simulink model "MNR"  (R2019b)
settings: Solver=FixedStepDiscrete  StartTime=0.0  StopTime=stop_time  RelTol=1e-3
InitFcn:
  | sm_callback_init
StopFcn:
  | sm_callback_stop
values from neighbouring files (symbols this model uses):
  mp = sm_init_avalon_signals(mp)    [sm_callback_init.m]    (also in sm_callback_stop.m = sm_stop_verify(mp))
libraries: simulink x1
settings Model: Creator=Ross  LastModifiedBy=trevor
settings DataIOCC: ReturnWorkspaceOutputs=off
settings OptimizationCC: BlockReduction=off  ConditionallyExecuteInputs=off  DefaultParameterBehavior=Inlined
settings DebuggingCC: ReadBeforeWriteMsg=DisableAll  WriteAfterWriteMsg=DisableAll  WriteAfterReadMsg=DisableAll  AlgebraicLoopMsg=error  MultiTaskDSMMsg=none  SingleTaskRateTransMsg=error  PregeneratedLibrarySubsystemCodeDiagnostic=none  ArithmeticOperatorsInVariantConditions=warning
settings HardwareCC: ProdBitPerPointer=32  ProdBitPerSizeT=32  ProdBitPerPtrDiffT=32  ProdLargestAtomicFloat=None  ProdIntDivRoundTo=Undefined  ProdEndianess=Unspecified  ProdWordSize=32  ProdHWDeviceType=ASIC/FPGA->ASIC/FPGA  TargetBitPerLong=64  TargetBitPerPointer=64  TargetBitPerSizeT=64  TargetBitPerPtrDiffT=64  TargetLongLongMode=on  TargetIntDivRoundTo=Zero  TargetEndianess=LittleEndian  TargetWordSize=64  TargetHWDeviceType=Custom Processor->MATLAB Host Computer  ProdEqTarget=off
settings ModelReferenceCC: UpdateModelReferenceTargets=IfOutOfDate
settings SFSimCC: SFSimEcho=off  SimUseLocalCustomCode=off  CustomCodeUndefinedFunction=UseInterfaceOnly
settings RTWCC: RTWUseLocalCustomCode=off

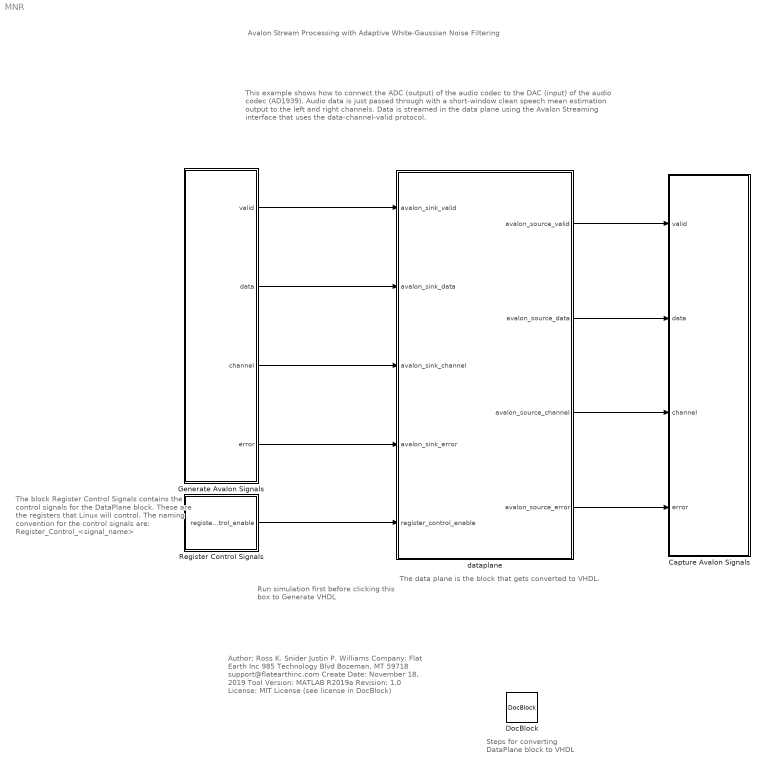
== system MNR ==
  note: The data plane is the block that gets converted to VHDL.
  note: Author:          Ross K. Snider
      |                      Justin P. Williams
      | Company:     Flat Earth Inc
      |                       985 Technology Blvd
      |                       Bozeman, MT 59718
      |                       support@flatearthinc.com
      | Create Date:  November 18, 2019
      | Tool Version:  MATLAB R2019a
      | Revision:        1.0
      | License:          MIT License (see license in DocBlock)
  note: This example shows how to connect the ADC (output) of the audio codec to the DAC (input) of the audio codec (AD1939). Audio data is just passed through with a short-window clean speech mean estimation output to the left and right channels. Data is streamed in the data plane using the Avalon Streaming interface that uses the data-channel-valid protocol.
  note: Steps for converting
      | DataPlane block
      | to VHDL
  note: Avalon Stream Processing
      | with Adaptive White-Gaussian Noise Filtering
  note: Run simulation first
      | before clicking this box to
      | Generate VHDL
  note: The block Register Control Signals contains
      | the control signals for the DataPlane block.
      | These are the registers that Linux will control.
      | The naming convention for the control
      | signals are:  Register_Control_<signal_name>
  Capture Avalon Signals : Subsystem
  DocBlock : simulink/Model-Wide Utilities/DocBlock  DocumentType=HTML
  Generate Avalon Signals : Subsystem
  Register Control Signals : Subsystem
  dataplane : Subsystem  TreatAsAtomicUnit=on
  wires:
  Generate Avalon Signals/2(data) -> dataplane/2(avalon_sink_data)
  Generate Avalon Signals/1(valid) -> dataplane/1(avalon_sink_valid)
  Generate Avalon Signals/3(channel) -> dataplane/3(avalon_sink_channel)
  Generate Avalon Signals/4(error) -> dataplane/4(avalon_sink_error)
  dataplane/2(avalon_source_data) -> Capture Avalon Signals/2(data)
  dataplane/1(avalon_source_valid) -> Capture Avalon Signals/1(valid)
  dataplane/3(avalon_source_channel) -> Capture Avalon Signals/3(channel)
  dataplane/4(avalon_source_error) -> Capture Avalon Signals/4(error)
  Register Control Signals/1(register_control_enable) -> dataplane/5(register_control_enable)

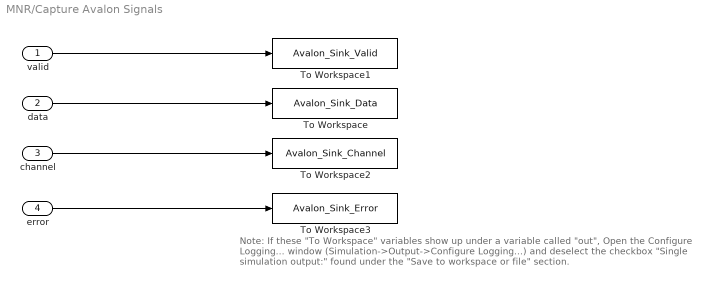
== system MNR/Capture Avalon Signals ==
  note: Note:  If these "To Workspace" variables show up under a variable called "out",
      | Open the Configure Logging... window (Simulation->Output->Configure Logging...)
      | and deselect the checkbox "Single simulation output:" found under the "Save to workspace or file" section.
  valid : Inport
  data : Inport  Port=2
  channel : Inport  Port=3
  error : Inport  Port=4
  To Workspace : ToWorkspace  VariableName=Avalon_Sink_Data  SaveFormat=Timeseries  SampleTime=-1
  To Workspace1 : ToWorkspace  VariableName=Avalon_Sink_Valid  SaveFormat=Timeseries  SampleTime=-1
  To Workspace2 : ToWorkspace  VariableName=Avalon_Sink_Channel  SaveFormat=Timeseries  SampleTime=-1
  To Workspace3 : ToWorkspace  VariableName=Avalon_Sink_Error  SaveFormat=Timeseries  SampleTime=-1
  wires:
  data/1 -> To Workspace/1
  valid/1 -> To Workspace1/1
  error/1 -> To Workspace3/1
  channel/1 -> To Workspace2/1

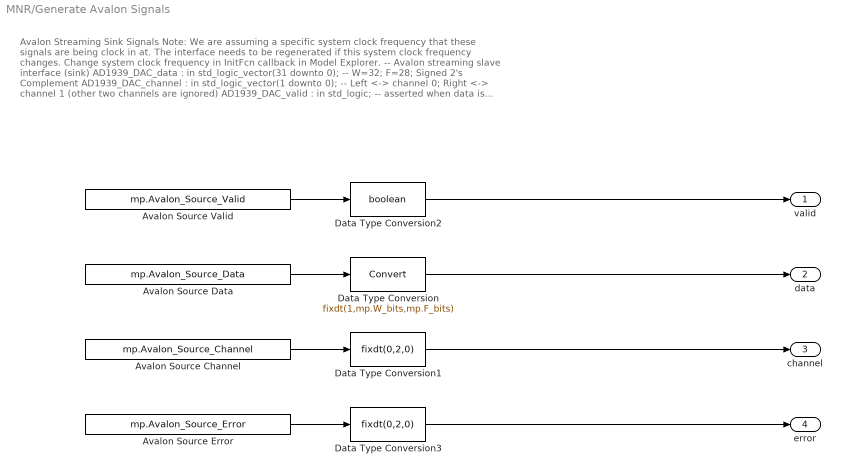
== system MNR/Generate Avalon Signals ==
  note: Avalon Streaming Sink Signals
      | Note: We are assuming a specific system clock frequency that these signals are being clock in at.
      | The interface needs to be regenerated if this system clock frequency changes. Change system clock frequency in InitFcn callback in Model Explorer.
      |
      | -- Avalon streaming slave interface (sink)
      | AD1939_DAC_data : in std_logic_vector(31 downto 0); -- W=32; F=28; Signed 2's Complement
      | AD1939_DAC_channel : in std_logic_vector(1 downto 0); -- Left <-> channel 0; Right <-> channel 1 (other two channels are ignored)
      | AD1939_DAC_valid : in std_logic; -- asserted when data is valid
      | AD1939_DAC_error : in std_logic_vector(1 downto 0) -- error channel is ignored, assumed to be error free at this point
      |
      | For more information on the data-channel-valid protocol, s ee chapter 5 in Intel's Avalon Interfaced Specification (p. 40) at https://www.intel.com/content/dam/www/programmable/us/en/pdfs/literature/manual/mnl_avalon_spec.pdf
  Avalon Source Channel : FromWorkspace  VariableName=mp.Avalon_Source_Channel  OutDataTypeStr=double  SampleTime=mp.Ts_system
  "Avalon Source Data " : FromWorkspace  VariableName=mp.Avalon_Source_Data  OutDataTypeStr=double  SampleTime=mp.Ts_system
  Avalon Source Error : FromWorkspace  VariableName=mp.Avalon_Source_Error  OutDataTypeStr=double  SampleTime=mp.Ts_system
  Avalon Source Valid : FromWorkspace  VariableName=mp.Avalon_Source_Valid  OutDataTypeStr=double  SampleTime=mp.Ts_system
  Data Type Conversion : DataTypeConversion  OutDataTypeStr=fixdt(1,mp.W_bits,mp.F_bits)
  Data Type Conversion1 : DataTypeConversion  OutDataTypeStr=fixdt(0,2,0)
  Data Type Conversion2 : DataTypeConversion  OutDataTypeStr=boolean
  Data Type Conversion3 : DataTypeConversion  OutDataTypeStr=fixdt(0,2,0)
  valid : Outport  VectorParamsAs1DForOutWhenUnconnected=off
  data : Outport  Port=2  VectorParamsAs1DForOutWhenUnconnected=off
  channel : Outport  Port=3  VectorParamsAs1DForOutWhenUnconnected=off
  error : Outport  Port=4  VectorParamsAs1DForOutWhenUnconnected=off
  wires:
  Data Type Conversion1/1 -> channel/1
  Data Type Conversion2/1 -> valid/1
  Avalon Source Error/1 -> Data Type Conversion3/1
  Data Type Conversion/1 -> data/1
  Avalon Source Valid/1 -> Data Type Conversion2/1
  Data Type Conversion3/1 -> error/1
  Avalon Source Channel/1 -> Data Type Conversion1/1
  "Avalon Source Data "/1 -> Data Type Conversion/1

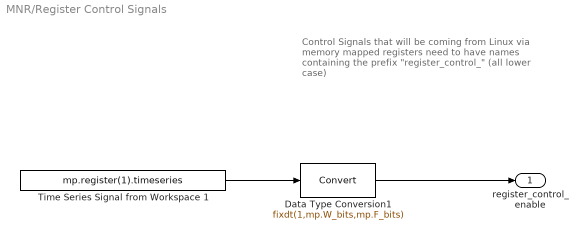
== system MNR/Register Control Signals ==
  note: Control Signals that will be coming from Linux via
      | memory mapped registers need to have names
      | containing the prefix "register_control_"
      | (all lower case)
  Data Type Conversion1 : DataTypeConversion  OutDataTypeStr=fixdt(1,mp.W_bits,mp.F_bits)
  Time Series Signal from Workspace 1 : FromWorkspace  VariableName=mp.register(1).timeseries  OutDataTypeStr=double  SampleTime=mp.Ts_system
  register_control_enable : Outport  VectorParamsAs1DForOutWhenUnconnected=off
  wires:
  Time Series Signal from Workspace 1/1 -> Data Type Conversion1/1
  Data Type Conversion1/1 -> register_control_enable/1

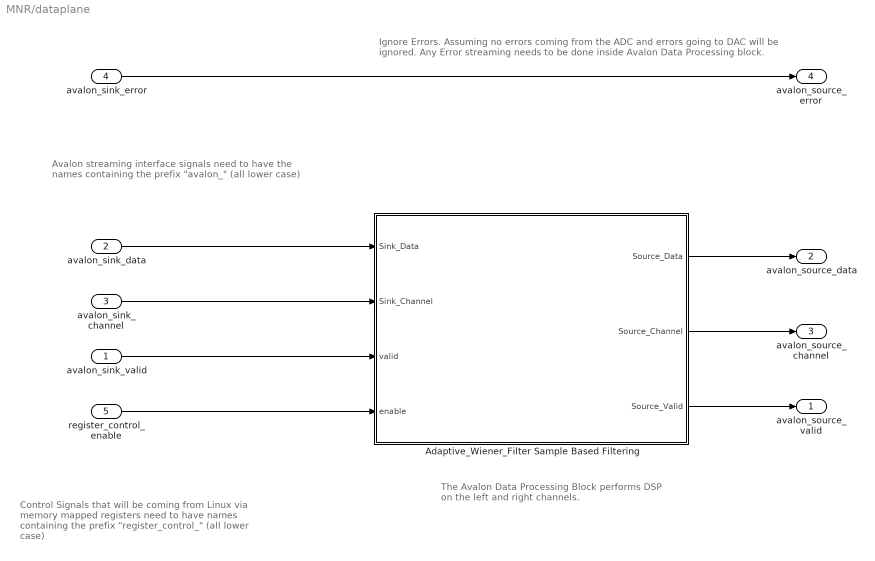
== system MNR/dataplane ==
  note: Control Signals that will be coming from Linux via
      | memory mapped registers need to have names
      | containing the prefix "register_control_"
      | (all lower case)
  note: The Avalon Data Processing Block
      | performs DSP on the left and right channels.
  note: Ignore Errors.
      | Assuming no errors coming from the ADC and errors going to DAC will be ignored.
      | Any Error streaming needs to be done inside Avalon Data Processing block.
  note: Avalon streaming interface signals need to have the
      | names containing the prefix "avalon_"
      | (all lower case)
  avalon_sink_valid : Inport
  avalon_sink_data : Inport  Port=2
  avalon_sink_channel : Inport  Port=3
  avalon_sink_error : Inport  Port=4
  register_control_enable : Inport  Port=5
  Adaptive_Wiener_Filter Sample Based Filtering : Subsystem
  avalon_source_valid : Outport  VectorParamsAs1DForOutWhenUnconnected=off
  avalon_source_data : Outport  Port=2  VectorParamsAs1DForOutWhenUnconnected=off
  avalon_source_channel : Outport  Port=3  VectorParamsAs1DForOutWhenUnconnected=off
  avalon_source_error : Outport  Port=4  VectorParamsAs1DForOutWhenUnconnected=off
  wires:
  avalon_sink_error/1 -> avalon_source_error/1
  Adaptive_Wiener_Filter Sample Based Filtering/1(Source_Data) -> avalon_source_data/1
  avalon_sink_data/1 -> Adaptive_Wiener_Filter Sample Based Filtering/1(Sink_Data)
  Adaptive_Wiener_Filter Sample Based Filtering/2(Source_Channel) -> avalon_source_channel/1
  avalon_sink_channel/1 -> Adaptive_Wiener_Filter Sample Based Filtering/2(Sink_Channel)
  register_control_enable/1 -> Adaptive_Wiener_Filter Sample Based Filtering/4(enable)
  avalon_sink_valid/1 -> Adaptive_Wiener_Filter Sample Based Filtering/3(valid)
  Adaptive_Wiener_Filter Sample Based Filtering/3(Source_Valid) -> avalon_source_valid/1

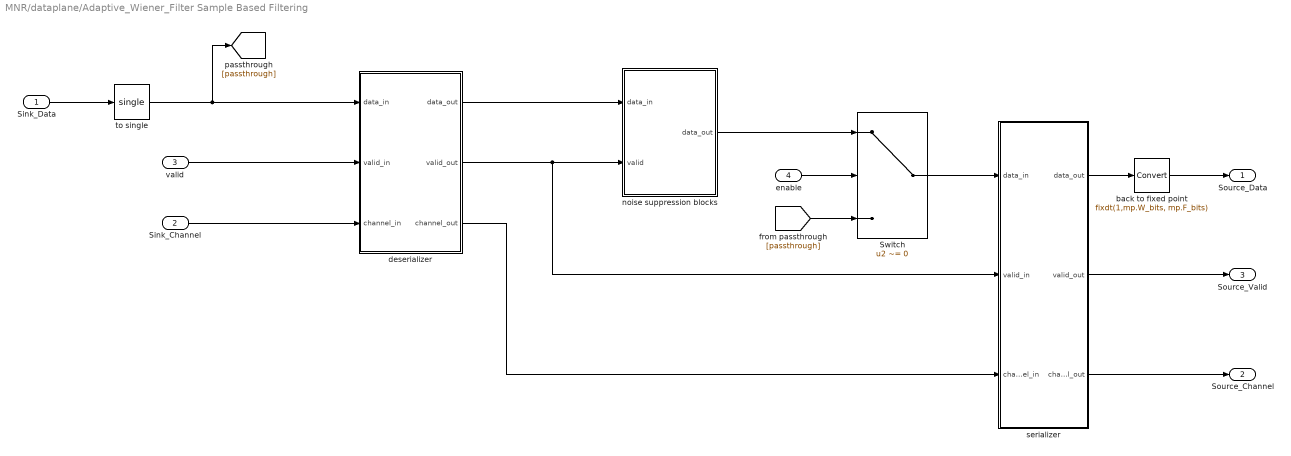
== system MNR/dataplane/Adaptive_Wiener_Filter Sample Based Filtering ==
  Sink_Data : Inport
  Sink_Channel : Inport  Port=2
  valid : Inport  Port=3
  enable : Inport  Port=4
  Switch : Switch  Criteria=u2 ~= 0  Threshold=1
  back to fixed point : DataTypeConversion  OutDataTypeStr=fixdt(1,mp.W_bits, mp.F_bits)  RndMeth=Nearest
  deserializer : MATLAB Function  TreatAsAtomicUnit=on
  noise suppression blocks : Subsystem  TreatAsAtomicUnit=on
  serializer : MATLAB Function  TreatAsAtomicUnit=on
  to single : DataTypeConversion  OutDataTypeStr=single  RndMeth=Nearest
  Source_Data : Outport  InitialOutput=0  VectorParamsAs1DForOutWhenUnconnected=off
  Source_Channel : Outport  Port=2  InitialOutput=0  VectorParamsAs1DForOutWhenUnconnected=off
  Source_Valid : Outport  Port=3  InitialOutput=0  VectorParamsAs1DForOutWhenUnconnected=off
  wires:
  enable/1 -> Switch/2
  to single/1 -> [passthrough], deserializer/1(data_in)
  valid/1 -> deserializer/2(valid_in)
  Sink_Channel/1 -> deserializer/3(channel_in)
  deserializer/2(valid_out) -> serializer/2(valid_in), noise suppression blocks/2(valid)
  deserializer/1(data_out) -> noise suppression blocks/1(data_in)
  noise suppression blocks/1(data_out) -> Switch/1
  [passthrough] -> Switch/3
  Sink_Data/1 -> to single/1
  back to fixed point/1 -> Source_Data/1
  serializer/1(data_out) -> back to fixed point/1
  Switch/1 -> serializer/1(data_in)
  serializer/3(channel_out) -> Source_Channel/1
  serializer/2(valid_out) -> Source_Valid/1
  deserializer/3(channel_out) -> serializer/3(channel_in)

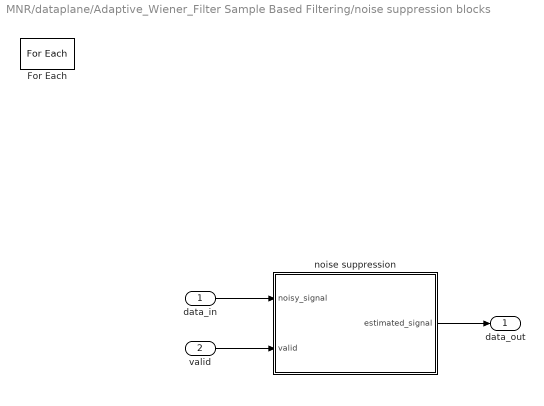
== system MNR/dataplane/Adaptive_Wiener_Filter Sample Based Filtering/noise suppression blocks ==
  data_in : Inport  Partition=on  PartitionDimension=1  PartitionWidth=1  PartitionOffset=0
  valid : Inport  Port=2
  For Each : ForEach  DisableCoverage=on
  noise suppression : Subsystem  TreatAsAtomicUnit=on
  data_out : Outport  ConcatenationDimension=1
  wires:
  noise suppression/1("estimated_signal ") -> data_out/1
  data_in/1 -> noise suppression/1(noisy_signal)
  valid/1 -> noise suppression/2(valid)

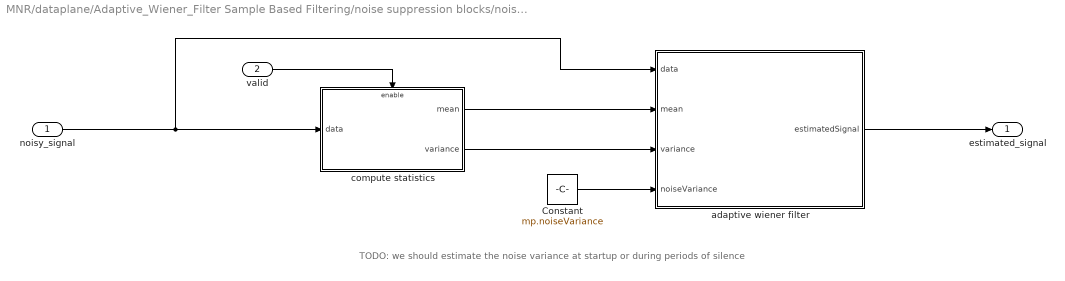
== system MNR/dataplane/Adaptive_Wiener_Filter Sample Based Filtering/noise suppression blocks/noise suppression ==
  note: TODO: we should estimate the noise variance at startup or during periods of silence
  noisy_signal : Inport
  valid : Inport  Port=2
  Constant : Constant  Value=mp.noiseVariance  SampleTime=-1
  adaptive wiener filter : MATLAB Function  TreatAsAtomicUnit=on
  compute statistics : Subsystem
  "estimated_signal " : Outport  InitialOutput=0  VectorParamsAs1DForOutWhenUnconnected=off
  wires:
  compute statistics/2(variance) -> adaptive wiener filter/3(variance)
  compute statistics/1(mean) -> adaptive wiener filter/2(mean)
  noisy_signal/1 -> adaptive wiener filter/1(data), compute statistics/1(data)
  valid/1 -> compute statistics/Enable
  adaptive wiener filter/1(estimatedSignal) -> "estimated_signal "/1
  Constant/1 -> adaptive wiener filter/4(noiseVariance)

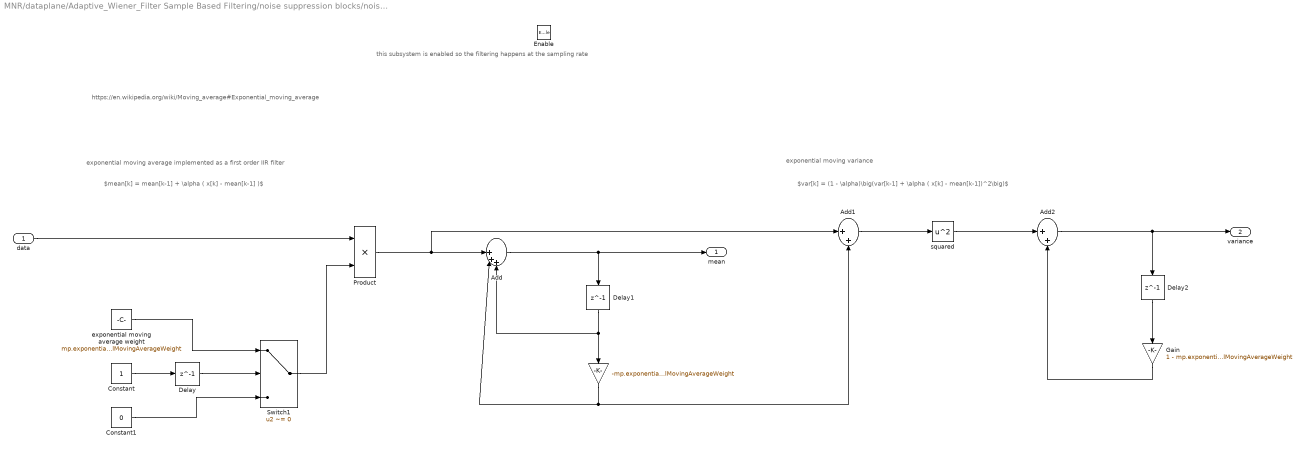
== system MNR/dataplane/Adaptive_Wiener_Filter Sample Based Filtering/noise suppression blocks/noise suppression/compute statistics ==
  note: https://en.wikipedia.org/wiki/Moving_average#Exponential_moving_average
  note: this subsystem is enabled so the filtering happens at the sampling rate
  note: $mean[k] = mean[k-1] + \alpha ( x[k] - mean[k-1] )$
  note: exponential moving variance
  note: exponential moving average implemented as a first order IIR filter
  note: $var[k] = (1 - \alpha)\big(var[k-1] + \alpha ( x[k] - mean[k-1])^2\big)$
  data : Inport
  Enable : EnablePort
  " " : Gain  Gain=-mp.exponentialMovingAverageWeight
  Add : Sum  Inputs=||+++
  Add1 : Sum  Inputs=|++
  Add2 : Sum  Inputs=|++
  Constant : Constant  OutDataTypeStr=boolean
  Constant1 : Constant  Value=0  OutDataTypeStr=single
  Delay : Delay  DelayLength=1  InitialCondition=0
  Delay1 : Delay  DelayLength=1  InitialCondition=0
  Delay2 : Delay  DelayLength=1  InitialCondition=0
  Gain : Gain  Gain=1 - mp.exponentialMovingAverageWeight
  Product : Product
  Switch1 : Switch  Criteria=u2 ~= 0
  exponential moving average weight : Constant  Value=mp.exponentialMovingAverageWeight
  squared : Math  Operator=square  RndMeth=Zero  SaturateOnIntegerOverflow=on
  mean : Outport
  variance : Outport  Port=2
  wires:
  Delay2/1 -> Gain/1
  Constant/1 -> Delay/1
  Switch1/1 -> Product/2
  Add2/1 -> variance/1, Delay2/1
  Add1/1 -> squared/1
  " "/1 -> Add/2, Add1/2
  Constant1/1 -> Switch1/3
  Delay/1 -> Switch1/2
  Product/1 -> Add1/1, Add/1
  Delay1/1 -> Add/3, " "/1
  exponential moving average weight/1 -> Switch1/1
  squared/1 -> Add2/1
  Add/1 -> mean/1, Delay1/1
  Gain/1 -> Add2/2
  data/1 -> Product/1

== matlab function MNR/dataplane/Adaptive_Wiener_Filter Sample Based Filtering/deserializer ==
  data: data_out output; valid_out output; data_in input; valid_in input; channel_in input; channel_out output
function [data_out, valid_out, channel_out] = deserialize(data_in, valid_in, channel_in)
%#codegen
persistent data_out_temp
persistent data_out_reg

% TODO: make determing the number of channels generic
if isempty(data_out_temp)
    data_out_temp = single(zeros(2, 1));
end
if isempty(data_out_reg)
    data_out_reg = single(zeros(2, 1));
end

valid_out = valid_in;
data_out = data_out_reg;
channel_out = channel_in;

if valid_in
    data_out_temp(channel_in + 1) = data_in;
    if channel_in == length(data_out_temp) - 1
%         valid_out = true;
        data_out_reg = data_out_temp;
    end
else
end

== matlab function MNR/dataplane/Adaptive_Wiener_Filter Sample Based Filtering/noise suppression blocks/noise suppression/adaptive wiener filter ==
  data: data input; estimatedSignal output; mean input; variance input; noiseVariance input
function estimatedSignal = adaptiveWienerFilter(data, mean, variance, noiseVariance)
%#codegen
estimatedSignal = mean + (variance / (variance + noiseVariance)) * (data - mean);

== matlab function MNR/dataplane/Adaptive_Wiener_Filter Sample Based Filtering/serializer ==
  data: data_out output; valid_out output; data_in input; valid_in input; channel_in input; channel_out output
function [data_out, valid_out, channel_out] = serialize(data_in, valid_in, channel_in)
%#codegen
persistent data_out_reg

if isempty(data_out_reg)
    data_out_reg = single(0);
end

if valid_in
    if channel_in == 0
        data_out_reg = data_in(1);
    elseif channel_in == 1
        data_out_reg = data_in(2);
    end
end

valid_out = valid_in;
channel_out = channel_in;
data_out = data_out_reg;
